simulink model "Assignment1Sim"  (R2020b)
settings: Solver=ode45  StartTime=0.0  StopTime=60  RelTol=1e-3
values from neighbouring files (symbols this model uses):
  a = 1    [Assignment1Mat.m]
  am = 1    [Assignment1Mat.m]
  b = 2    [Assignment1Mat.m]
  sinAmp = 0    [Assignment1Mat.m]
  sinFreq = (2*pi)/(24*3600)    (= 7.27220521664e-05)    [Assignment1Mat.m]
libraries: simulink x2
settings Model: Creator=Paolo  LastModifiedBy=Paolo

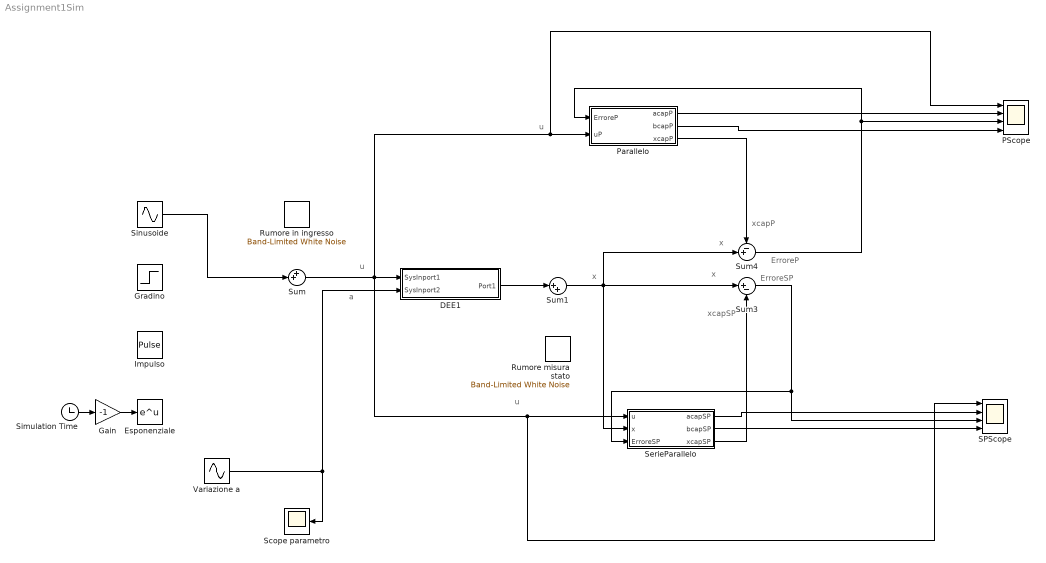
== system Assignment1Sim ==
  note: ErroreP
  note: x
  note: xcapP
  note: ErroreSP
  note: xcapSP
  note: x
  note: u
  note: u
  note: a
  note: u
  note: x
  "DEE1 " : Subsystem  mask(Differential Equation Editor (DEE)){}
      settings: OpenFcn=diffeqed
      mask Display: disp('Sistema')
  Esponenziale : Math  SaturateOnIntegerOverflow=on
  Gain : Gain  Gain=-1
  Gradino : Step  SampleTime=0
  Impulso : DiscretePulseGenerator  PulseType=Time based  Amplitude=10  Period=120  PulseWidth=5  PhaseDelay=1
  PScope : Scope  NumInputPorts=4
  Parallelo : Subsystem
  Rumore in ingresso : simulink/Sources/Band-Limited White Noise  Cov=[0.001]  Ts=0.1  seed=[2230]
  Rumore misura stato : simulink/Sources/Band-Limited White Noise  Cov=[0.1]  Ts=0.1  seed=[58]
  SPScope : Scope  NumInputPorts=4
  Scope parametro : Scope
  SerieParallelo : Subsystem
  Simulation Time : Clock
  Sinusoide : Sin  SampleTime=0
  Sum : Sum  Inputs=++|
  Sum1 : Sum  Inputs=|++
  Sum3 : Sum  Inputs=|+-
  Sum4 : Sum  Inputs=-+|
  Variazione a : Sin  Amplitude=sinAmp  Bias=a  Frequency=sinFreq  SampleTime=0
  wires:
  Simulation Time/1 -> Gain/1
  Gain/1 -> Esponenziale/1
  Sum/1 -> SPScope/1, SerieParallelo/1(u), PScope/1, Parallelo/2(uP), "DEE1 "/1(SysInport1)
  "DEE1 "/1(Port1) -> Sum1/1
  Sum1/1 -> SerieParallelo/2(x), Sum3/1, Sum4/2
  Sum3/1 -> SPScope/3, SerieParallelo/3(ErroreSP)
  Sum4/1 -> PScope/3, Parallelo/1(ErroreP)
  Parallelo/1(acapP) -> PScope/2
  Parallelo/3(xcapP) -> Sum4/1
  SerieParallelo/3(xcapSP) -> Sum3/2
  SerieParallelo/1(acapSP) -> SPScope/2
  Parallelo/2(bcapP) -> PScope/4
  SerieParallelo/2(bcapSP) -> SPScope/4
  Variazione a/1 -> Scope parametro/1, "DEE1 "/2(SysInport2)
  Sinusoide/1 -> Sum/2

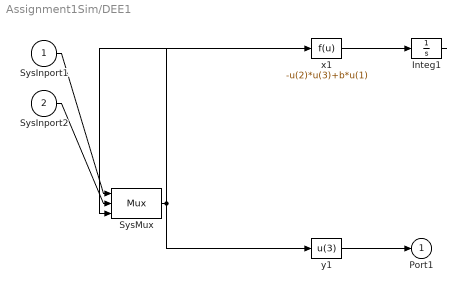
== system Assignment1Sim/DEE1  ==
  SysInport1 : Inport
  SysInport2 : Inport  Port=2
  Integ1 : Integrator
  SysMux : Mux  Inputs=3
  x1 : Fcn  Expr=-u(2)*u(3)+b*u(1)
  y1 : Fcn  Expr=u(3)
  Port1 : Outport
  wires:
  SysInport1/1 -> SysMux/1
  SysInport2/1 -> SysMux/2
  SysMux/1 -> x1/1, y1/1
  x1/1 -> Integ1/1
  Integ1/1 -> SysMux/3
  y1/1 -> Port1/1

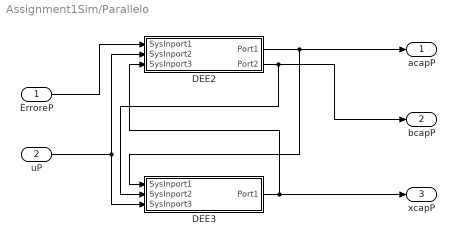
== system Assignment1Sim/Parallelo ==
  ErroreP : Inport
  uP : Inport  Port=2
  DEE2 : Subsystem  mask(Differential Equation Editor (DEE)){}
      settings: OpenFcn=diffeqed
      mask Display: disp('Stimatore')
  DEE3 : Subsystem  mask(Differential Equation Editor (DEE)){}
      settings: OpenFcn=diffeqed
      mask Display: disp('Sistema Stimato')
  acapP : Outport
  bcapP : Outport  Port=2
  xcapP : Outport  Port=3
  wires:
  DEE2/1(Port1) -> DEE3/1(SysInport1), acapP/1
  DEE2/2(Port2) -> DEE3/2(SysInport2), bcapP/1
  DEE3/1(Port1) -> DEE2/3(SysInport3), xcapP/1
  ErroreP/1 -> DEE2/1(SysInport1)
  uP/1 -> DEE3/3(SysInport3), DEE2/2(SysInport2)

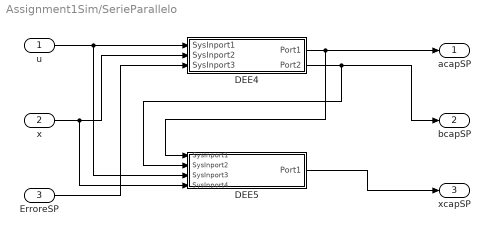
== system Assignment1Sim/SerieParallelo ==
  u : Inport
  x : Inport  Port=2
  ErroreSP : Inport  Port=3
  DEE4 : Subsystem  mask(Differential Equation Editor (DEE)){}
      settings: OpenFcn=diffeqed
      mask Display: disp('Stimatore')
  DEE5 : Subsystem  mask(Differential Equation Editor (DEE)){}
      settings: OpenFcn=diffeqed
      mask Display: disp('Sistema Stimato')
  acapSP : Outport
  bcapSP : Outport  Port=2
  xcapSP : Outport  Port=3
  wires:
  u/1 -> DEE5/3(SysInport3), DEE4/1(SysInport1)
  x/1 -> DEE5/4(SysInport4), DEE4/2(SysInport2)
  ErroreSP/1 -> DEE4/3(SysInport3)
  DEE4/2(Port2) -> DEE5/2(SysInport2), bcapSP/1
  DEE4/1(Port1) -> DEE5/1(SysInport1), acapSP/1
  DEE5/1(Port1) -> xcapSP/1

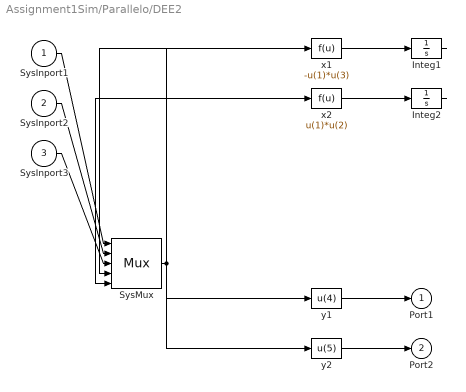
== system Assignment1Sim/Parallelo/DEE2 ==
  SysInport1 : Inport
  SysInport2 : Inport  Port=2
  SysInport3 : Inport  Port=3
  Integ1 : Integrator
  Integ2 : Integrator
  SysMux : Mux  Inputs=5
  x1 : Fcn  Expr=-u(1)*u(3)
  x2 : Fcn  Expr=u(1)*u(2)
  y1 : Fcn  Expr=u(4)
  y2 : Fcn  Expr=u(5)
  Port1 : Outport
  Port2 : Outport  Port=2
  wires:
  SysInport1/1 -> SysMux/1
  SysInport2/1 -> SysMux/2
  SysInport3/1 -> SysMux/3
  SysMux/1 -> x1/1, x2/1, y1/1, y2/1
  x1/1 -> Integ1/1
  Integ1/1 -> SysMux/4
  x2/1 -> Integ2/1
  Integ2/1 -> SysMux/5
  y1/1 -> Port1/1
  y2/1 -> Port2/1

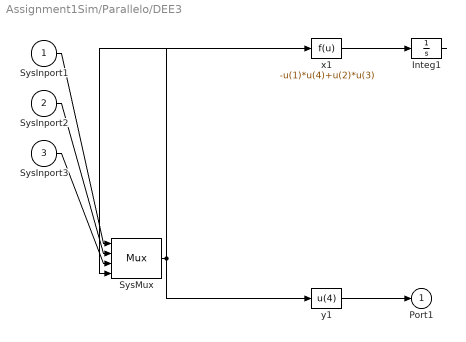
== system Assignment1Sim/Parallelo/DEE3 ==
  SysInport1 : Inport
  SysInport2 : Inport  Port=2
  SysInport3 : Inport  Port=3
  Integ1 : Integrator
  SysMux : Mux
  x1 : Fcn  Expr=-u(1)*u(4)+u(2)*u(3)
  y1 : Fcn  Expr=u(4)
  Port1 : Outport
  wires:
  SysInport1/1 -> SysMux/1
  SysInport2/1 -> SysMux/2
  SysInport3/1 -> SysMux/3
  SysMux/1 -> x1/1, y1/1
  x1/1 -> Integ1/1
  Integ1/1 -> SysMux/4
  y1/1 -> Port1/1

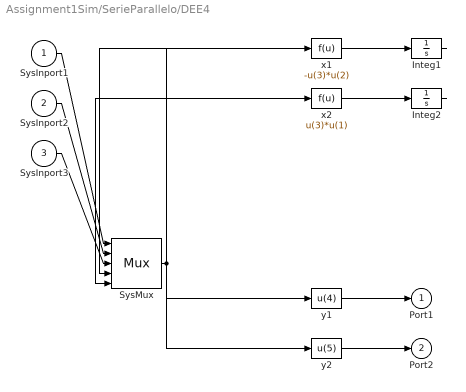
== system Assignment1Sim/SerieParallelo/DEE4 ==
  SysInport1 : Inport
  SysInport2 : Inport  Port=2
  SysInport3 : Inport  Port=3
  Integ1 : Integrator
  Integ2 : Integrator
  SysMux : Mux  Inputs=5
  x1 : Fcn  Expr=-u(3)*u(2)
  x2 : Fcn  Expr=u(3)*u(1)
  y1 : Fcn  Expr=u(4)
  y2 : Fcn  Expr=u(5)
  Port1 : Outport
  Port2 : Outport  Port=2
  wires:
  SysInport1/1 -> SysMux/1
  SysInport2/1 -> SysMux/2
  SysInport3/1 -> SysMux/3
  SysMux/1 -> x1/1, x2/1, y1/1, y2/1
  x1/1 -> Integ1/1
  Integ1/1 -> SysMux/4
  x2/1 -> Integ2/1
  Integ2/1 -> SysMux/5
  y1/1 -> Port1/1
  y2/1 -> Port2/1

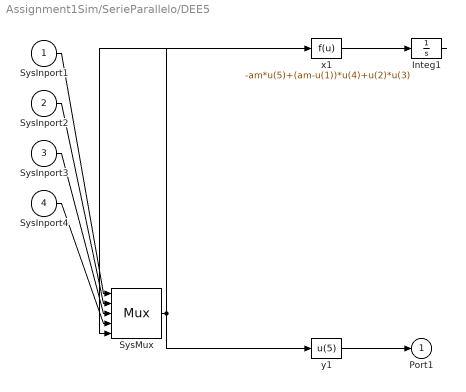
== system Assignment1Sim/SerieParallelo/DEE5 ==
  SysInport1 : Inport
  SysInport2 : Inport  Port=2
  SysInport3 : Inport  Port=3
  SysInport4 : Inport  Port=4
  Integ1 : Integrator
  SysMux : Mux  Inputs=5
  x1 : Fcn  Expr=-am*u(5)+(am-u(1))*u(4)+u(2)*u(3)
  y1 : Fcn  Expr=u(5)
  Port1 : Outport
  wires:
  SysInport1/1 -> SysMux/1
  SysInport2/1 -> SysMux/2
  SysInport3/1 -> SysMux/3
  SysInport4/1 -> SysMux/4
  SysMux/1 -> x1/1, y1/1
  x1/1 -> Integ1/1
  Integ1/1 -> SysMux/5
  y1/1 -> Port1/1
